simulink model "plotter_taut_constraint"  (R2025a)
settings: Solver=VariableStepAuto  StartTime=0.0  StopTime=6  RelTol=1e-3
values from neighbouring files (symbols this model uses):
  alfa = cos(0.34906585)    [parameters.m]
  B_m = 0.000002    (= 2e-06)    [parameters.m]
  g = 9.8    [parameters.m]
  Gr = 1/30    (= 0.0333333333333)    [parameters.m]
  J_m = 0.000004    (= 4e-06)    [parameters.m]
  K_t = 0.009    [parameters.m]
  L = 0.3    [cinematic_sim.m]    (also in parameters.m)
  L_a = 0.0023    [parameters.m]
  m = 0.1    [parameters.m]
  R = 0.017    [parameters.m]
  R_a = 2.182    [parameters.m]
libraries: slpidlib x2
settings Model: Creator=bruno  LastModifiedBy=bruno

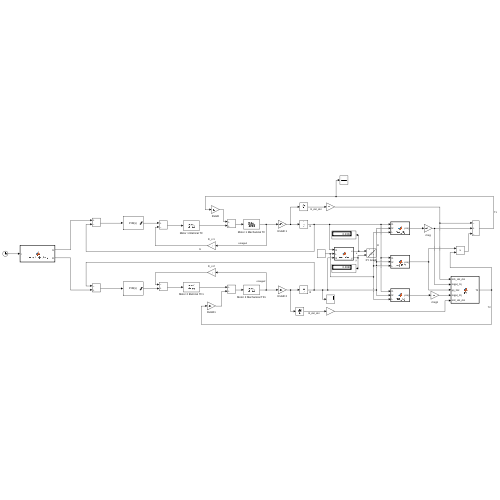
[thumbnail: Simulink's stored preview of the top-level diagram]
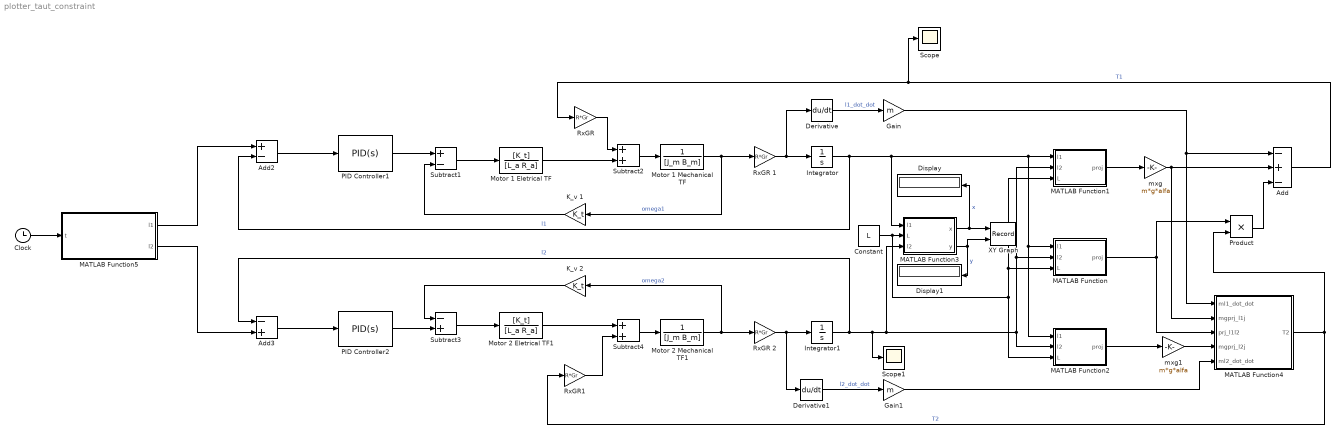
== system plotter_taut_constraint ==
  Add : Sum  Inputs=-+-
  Add2 : Sum  Inputs=+-
  Add3 : Sum  Inputs=-+
  Clock : Clock
      settings: Decimation=1000
  Constant : Constant  Value=L
  Derivative : Derivative
  Derivative1 : Derivative
  Display : Display
  Display1 : Display
  Gain : Gain  Gain=m
  Gain1 : Gain  Gain=m
  Integrator : Integrator  InitialCondition=0.461411
  Integrator1 : Integrator  InitialCondition=0.406079
  K_v 1 : Gain  Gain=K_t
  K_v 2 : Gain  Gain=K_t
  MATLAB Function : MATLAB Function  TreatAsAtomicUnit=on
  MATLAB Function1 : MATLAB Function  TreatAsAtomicUnit=on
  MATLAB Function2 : MATLAB Function  TreatAsAtomicUnit=on
  MATLAB Function3 : MATLAB Function  TreatAsAtomicUnit=on
  MATLAB Function4 : MATLAB Function  TreatAsAtomicUnit=on
  MATLAB Function5 : MATLAB Function  TreatAsAtomicUnit=on
  Motor 1 Eletrical TF : TransferFcn  Numerator=[K_t]  Denominator=[L_a R_a]
  Motor 1 Mechanical TF : TransferFcn  Denominator=[J_m B_m]
  Motor 2 Eletrical TF1 : TransferFcn  Numerator=[K_t]  Denominator=[L_a R_a]
  Motor 2 Mechanical TF1 : TransferFcn  Denominator=[J_m B_m]
  PID Controller1 : slpidlib/PID Controller  Controller=PID  Form=Parallel  TimeDomain=Continuous-time  UseExternalTs=off  SampleTime=-1  IntegratorMethod=Forward Euler  FilterMethod=Forward Euler  ControllerParametersSource=internal  P=5109.01806071816  I=6474.67483762337  UseKiTs=off  D=175.0621895201  UseExternalDerivativeSource=off  N=17340.6505292231  UseFilter=on  TunerSelectOption=Transfer Function Based (PID Tuner App)  InitialConditionSource=internal  InitialConditionForIntegrator=0  InitialConditionForFilter=0  DifferentiatorICPrevScaledInput=0  ExternalReset=none  TrackingMode=off  Kt=1  LimitOutput=on  SatLimitsSource=internal  UpperSaturationLimit=12  LowerSaturationLimit=-12  LinearizeAsGain=on  AntiWindupMode=none  Kb=1  LimitIntegrator=off  UpperIntegratorSaturationLimit=inf  LowerIntegratorSaturationLimit=-inf  POutMin=[]  POutMax=[]  IOutMin=[]  IOutMax=[]  DOutMin=[]  DOutMax=[]  NOutMin=[]  NOutMax=[]  SumOutMin=[]  SumOutMax=[]  SaturationOutMin=[]  SaturationOutMax=[]  PParamMin=[]  PParamMax=[]  IParamMin=[]  IParamMax=[]  DParamMin=[]  DParamMax=[]  NParamMin=[]  NParamMax=[]  KbParamMin=[]  KbParamMax=[]  KtParamMin=[]  KtParamMax=[]  KbOutMin=[]  KbOutMax=[]  KtOutMin=[]  KtOutMax=[]  IntegratorOutMin=[]  IntegratorOutMax=[]  FilterOutMin=[]  FilterOutMax=[]  SumI1OutMin=[]  SumI1OutMax=[]  SumI2OutMin=[]  SumI2OutMax=[]  SumI3OutMin=[]  SumI3OutMax=[]  SumI4OutMin=[]  SumI4OutMax=[]  SumDOutMin=[]  SumDOutMax=[]  DifferentiatorOutMin=[]  DifferentiatorOutMax=[]  FilterDiffOutCoefMin=[]  FilterDiffOutCoefMax=[]  ReciprocalOutMin=[]  ReciprocalOutMax=[]  SumDenOutMin=[]  SumDenOutMax=[]  SumNumOutMin=[]  SumNumOutMax=[]  DivideOutMin=[]  DivideOutMax=[]  UdiffTsProdOutMin=[]  UdiffTsProdOutMax=[]  NTsProdOutMin=[]  NTsProdOutMax=[]  UintegralTsProdOutMin=[]  UintegralTsProdOutMax=[]  UngainTsProdOutMin=[]  UngainTsProdOutMax=[]  ClampingZeroOutDataTypeStr=Inherit: Inherit via back propagation  ClampingZeroOutMin=[]  ClampingZeroOutMax=[]  FilterDenConstantOutDataTypeStr=Inherit: Inherit via back propagation  FilterDenConstantOutMin=[]  FilterDenConstantOutMax=[]  PCopyOutDataTypeStr=Inherit: Inherit via back propagation  PCopyOutMin=[]  PCopyOutMax=[]  NCopyOutDataTypeStr=Inherit: Inherit via back propagation  NCopyOutMin=[]  NCopyOutMax=[]  IntegratorContinuousStateAttributes=''  IntegratorStateMustResolveToSignalObject=off  IntegratorRTWStateStorageClass=Auto  FilterContinuousStateAttributes=''  FilterStateMustResolveToSignalObject=off  FilterRTWStateStorageClass=Auto  ParallelPVariant=InternalParameters  IdealPVariant=Disabled  IVariant=InternalParameters  DVariant=InternalParameters  IntegratorVariant=Continuous  SatVariant=Enabled  AWVariant=Passthrough  PCopyVariant=Disabled  TRVariant=Disabled  FdbkBlocksVariant=Forward  IdealPFdbkVariant=Disabled  SatFdbkVariant=Disabled  DerivativeFilterVariant=ContFilter  NVariant=InternalParameters  NCopyVariant=Disabled  FilterICVariant=InternalICsFilter  IntegratorICVariant=InternalICs  ExternalResetVariant=Disabled  TRSumVariant=Passthrough  SumFdbkVariant=Disabled  SumVariant=Sum_PID  TsampFilterVariant=InternalTs  TsampNgainVariant=Passthrough  TsampIntegralVariant=Disabled_SignalSpec  ExternalSaturationOutDataTypeStr=Inherit: Same as second input  DerivativeSourceVariant=ErrorSignal  PreIntVariant=InternalPreInt
  PID Controller2 : slpidlib/PID Controller  Controller=PID  Form=Parallel  TimeDomain=Continuous-time  UseExternalTs=off  SampleTime=-1  IntegratorMethod=Forward Euler  FilterMethod=Forward Euler  ControllerParametersSource=internal  P=5109.01806071816  I=6474.67483762337  UseKiTs=off  D=175.0621895201  UseExternalDerivativeSource=off  N=17340.6505292231  UseFilter=on  TunerSelectOption=Transfer Function Based (PID Tuner App)  InitialConditionSource=internal  InitialConditionForIntegrator=0  InitialConditionForFilter=0  DifferentiatorICPrevScaledInput=0  ExternalReset=none  TrackingMode=off  Kt=1  LimitOutput=on  SatLimitsSource=internal  UpperSaturationLimit=12  LowerSaturationLimit=-12  LinearizeAsGain=on  AntiWindupMode=none  Kb=1  LimitIntegrator=off  UpperIntegratorSaturationLimit=inf  LowerIntegratorSaturationLimit=-inf  POutMin=[]  POutMax=[]  IOutMin=[]  IOutMax=[]  DOutMin=[]  DOutMax=[]  NOutMin=[]  NOutMax=[]  SumOutMin=[]  SumOutMax=[]  SaturationOutMin=[]  SaturationOutMax=[]  PParamMin=[]  PParamMax=[]  IParamMin=[]  IParamMax=[]  DParamMin=[]  DParamMax=[]  NParamMin=[]  NParamMax=[]  KbParamMin=[]  KbParamMax=[]  KtParamMin=[]  KtParamMax=[]  KbOutMin=[]  KbOutMax=[]  KtOutMin=[]  KtOutMax=[]  IntegratorOutMin=[]  IntegratorOutMax=[]  FilterOutMin=[]  FilterOutMax=[]  SumI1OutMin=[]  SumI1OutMax=[]  SumI2OutMin=[]  SumI2OutMax=[]  SumI3OutMin=[]  SumI3OutMax=[]  SumI4OutMin=[]  SumI4OutMax=[]  SumDOutMin=[]  SumDOutMax=[]  DifferentiatorOutMin=[]  DifferentiatorOutMax=[]  FilterDiffOutCoefMin=[]  FilterDiffOutCoefMax=[]  ReciprocalOutMin=[]  ReciprocalOutMax=[]  SumDenOutMin=[]  SumDenOutMax=[]  SumNumOutMin=[]  SumNumOutMax=[]  DivideOutMin=[]  DivideOutMax=[]  UdiffTsProdOutMin=[]  UdiffTsProdOutMax=[]  NTsProdOutMin=[]  NTsProdOutMax=[]  UintegralTsProdOutMin=[]  UintegralTsProdOutMax=[]  UngainTsProdOutMin=[]  UngainTsProdOutMax=[]  ClampingZeroOutDataTypeStr=Inherit: Inherit via back propagation  ClampingZeroOutMin=[]  ClampingZeroOutMax=[]  FilterDenConstantOutDataTypeStr=Inherit: Inherit via back propagation  FilterDenConstantOutMin=[]  FilterDenConstantOutMax=[]  PCopyOutDataTypeStr=Inherit: Inherit via back propagation  PCopyOutMin=[]  PCopyOutMax=[]  NCopyOutDataTypeStr=Inherit: Inherit via back propagation  NCopyOutMin=[]  NCopyOutMax=[]  IntegratorContinuousStateAttributes=''  IntegratorStateMustResolveToSignalObject=off  IntegratorRTWStateStorageClass=Auto  FilterContinuousStateAttributes=''  FilterStateMustResolveToSignalObject=off  FilterRTWStateStorageClass=Auto  ParallelPVariant=InternalParameters  IdealPVariant=Disabled  IVariant=InternalParameters  DVariant=InternalParameters  IntegratorVariant=Continuous  SatVariant=Enabled  AWVariant=Passthrough  PCopyVariant=Disabled  TRVariant=Disabled  FdbkBlocksVariant=Forward  IdealPFdbkVariant=Disabled  SatFdbkVariant=Disabled  DerivativeFilterVariant=ContFilter  NVariant=InternalParameters  NCopyVariant=Disabled  FilterICVariant=InternalICsFilter  IntegratorICVariant=InternalICs  ExternalResetVariant=Disabled  TRSumVariant=Passthrough  SumFdbkVariant=Disabled  SumVariant=Sum_PID  TsampFilterVariant=InternalTs  TsampNgainVariant=Passthrough  TsampIntegralVariant=Disabled_SignalSpec  ExternalSaturationOutDataTypeStr=Inherit: Same as second input  DerivativeSourceVariant=ErrorSignal  PreIntVariant=InternalPreInt
  Product : Product
  RxGR : Gain  Gain=R*Gr
  RxGR 1 : Gain  Gain=R*Gr
  RxGR 2 : Gain  Gain=R*Gr
  RxGR1 : Gain  Gain=R*Gr
  Scope : Scope
      settings: ActiveDisplayYMinimum=0.083131724548446431  ActiveDisplayYMaximum=0.66068166204181777
  Scope1 : Scope
      settings: ActiveDisplayYMinimum=-1  ActiveDisplayYMaximum=1
  Subtract1 : Sum  Inputs=+-
  Subtract2 : Sum
  Subtract3 : Sum  Inputs=-+
  Subtract4 : Sum
  XY Graph : Record  NumPorts=2.0  FileSettingsInternal="{\"entries\":[{\"content\":{\"excelSettings\":{\"content\":{},\"type\":\"Streamout.ExcelSettings\"},\"parquetSettings\":{\"content\":{},\"type\":\"Streamout.ParquetSettings\"}},\"type\":\"Streamout.FileSettingStorage\",\"uuid\":\"\"}],\"packageUris\":[\"http:\\/\\/schema.mathworks.com\\/mf0\\/streamout_blocks\\/R2020a\"],\"version\":\"1.0\"}"  FrameSettings=[0, 0]  Layout=[1 1]  SignalsInternal="{\"entries\":[{\"content\":{\"signals\":[{\"content\":{\"blockPath\":[],\"dimensions\":[1],\"domain\":\"\",\"lineColor\":\"#a2142f\",\"plots\":[ 1 ],\"port\":1,\"sid\":[\"\"],\"signalID\":1,\"signalName\":\"x\"},\"type\":\"RecordBlkView.Signal\",\"uuid\":\"\"},{\"content\":{\"blockPath\":[],\"dimensions\":[1],\"domain\":\"\",\"lineColor\":\"#139fff\",\"plots\":[ 1 ],\"port\":2,\"sid\":[\"\"],\"signalID\":2,\"signalName\":\"y\"},\"type\":\"RecordBlkView.Signal\",\"uuid\":\"\"}]},\"type\":\"RecordBlkView.InputSignals\",\"uuid\":\"\"}],\"packageUris\":[\"http:\\/\\/schema.mathworks.com\\/mf0\\/streamout_blocks\\/R2020a\"],\"version\":\"1.0\"}"  VisualizationBindings="{\"xyplotplugin\":{\"info\":[{\"series\":[{\"bindingParametersList\":[{\"parameter\":\"X-Axis\",\"signalID\":1,\"signalName\":\"x\"},{\"parameter\":\"Y-Axis\",\"signalID\":2,\"signalName\":\"y\"}],\"seriesID\":0}],\"subplotID\":1}]}}"  CompatibilityTag=XY
  mxg : Gain  Gain=m*g*alfa
  mxg1 : Gain  Gain=m*g*alfa
  wires:
  Motor 1 Eletrical TF/1 -> Subtract2/2
  Subtract2/1 -> Motor 1 Mechanical TF/1
  RxGR/1 -> Subtract2/1
  Motor 1 Mechanical TF/1 -> RxGR 1/1, K_v 1/1  "omega1"
  Subtract1/1 -> Motor 1 Eletrical TF/1
  PID Controller1/1 -> Subtract1/1
  RxGR 1/1 -> Derivative/1, Integrator/1
  K_v 1/1 -> Subtract1/2
  Derivative/1 -> Gain/1  "l1_dot_dot"
  Derivative1/1 -> Gain1/1  "l2_dot_dot"
  Motor 2 Mechanical TF1/1 -> RxGR 2/1, K_v 2/1  "omega2"
  Motor 2 Eletrical TF1/1 -> Subtract4/1
  RxGR 2/1 -> Derivative1/1, Integrator1/1
  Subtract4/1 -> Motor 2 Mechanical TF1/1
  Subtract3/1 -> Motor 2 Eletrical TF1/1
  K_v 2/1 -> Subtract3/1
  RxGR1/1 -> Subtract4/2
  Integrator/1 -> Add2/2, MATLAB Function3/1(l1), MATLAB Function2/1(l1), MATLAB Function/1(l1), MATLAB Function1/1(l1)  "l1"
  Integrator1/1 -> Add3/1, Scope1/1, MATLAB Function1/2(l2), MATLAB Function/2(l2), MATLAB Function2/2(l2), MATLAB Function3/3(l2)  "l2"
  Constant/1 -> MATLAB Function1/3(L), MATLAB Function/3(L), MATLAB Function2/3(L), MATLAB Function3/2(L)
  MATLAB Function1/1(proj) -> mxg/1
  MATLAB Function/1(proj) -> Product/1, MATLAB Function4/3(prj_l1l2)
  Product/1 -> Add/3
  mxg/1 -> Add/2, MATLAB Function4/2(mgprj_l1j)
  Gain/1 -> MATLAB Function4/1(ml1_dot_dot), Add/1
  Add/1 -> Scope/1, RxGR/1  "T1"
  MATLAB Function2/1(proj) -> mxg1/1
  mxg1/1 -> MATLAB Function4/4(mgprj_l2j)
  MATLAB Function4/1(T2) -> RxGR1/1, Product/2  "T2"
  MATLAB Function3/1(x) -> XY Graph/1, Display/1  "x"
  MATLAB Function3/2(y) -> XY Graph/2, Display1/1  "y"
  Gain1/1 -> MATLAB Function4/5(ml2_dot_dot)
  PID Controller2/1 -> Subtract3/2
  Add3/1 -> PID Controller2/1
  Add2/1 -> PID Controller1/1
  Clock/1 -> MATLAB Function5/1(t)
  MATLAB Function5/1(l1) -> Add2/1
  MATLAB Function5/2(l2) -> Add3/2

== matlab function plotter_taut_constraint/MATLAB Function1 ==
  data: l1 input; proj output; l2 input; L input
function proj = proj_l1j(l1,l2,L)

proj = sqrt(l1^2-(L^2+l1^2-l2^2)^2/(4*L^2))/l1;

== matlab function plotter_taut_constraint/MATLAB Function ==
  data: l1 input; proj output; l2 input; L input
function proj = proj_l1l2(l1,l2,L)

proj = (l1^2 + l2^2 + L^2)/(2*l1*l2);

== matlab function plotter_taut_constraint/MATLAB Function2 ==
  data: l1 input; proj output; l2 input; L input
function proj = proj_l2j(l1,l2,L)

proj = sqrt(l1^2-(L^2+l1^2-l2^2)^2/(4*L^2))/l2;

== matlab function plotter_taut_constraint/MATLAB Function3 ==
  data: x output; l1 input; L input; y output; l2 input
function [x,y]= rev_kin(l1,L,l2)

x = (L^2+l1^2-l2^2)/(2*L);
y = sqrt(l1^2 - x^2);

== matlab function plotter_taut_constraint/MATLAB Function4 ==
  data: ml1_dot_dot input; mgprj_l1j input; prj_l1l2 input; mgprj_l2j input; T2 output; ml2_dot_dot input
function T2 = T2(ml1_dot_dot,mgprj_l1j,prj_l1l2,mgprj_l2j,ml2_dot_dot)

T2 = (-ml2_dot_dot + ml1_dot_dot*prj_l1l2 - mgprj_l1j*prj_l1l2 + mgprj_l2j)/(1-prj_l1l2^2);

== matlab function plotter_taut_constraint/MATLAB Function5 ==
  data: l1 output; l2 output; t input
function [l1, l2] = circle_trajectory(t)
% Generate (x, y) circular trajectory given time t

% Parameters
T = 6;           % Period (seconds)
r = 0.08;        % Radius (meters)
x0 = 0.15;       % Center x (meters)
y0 = 0.4;        % Center y (meters)
L = 0.3;

% Equations
angle = 2 * pi * t / T;
x = r * cos(angle) + x0;
y = r * sin(angle) + y0;
l1 = sqrt(x^2 + y^2);
l2 = sqrt((L - x)^2 + y^2);
